simulink model "linear_Plant"  (Simulink 8.1)
settings: Solver=ode4  StartTime=0.0  StopTime=10  FixedStep=0.001  RelTol=1e-3
values from neighbouring files (symbols this model uses):
  a_m = -4    [MRAC_script.m]
  a_p = 1    [MRAC_script.m]
  Gamma = eye(6)*2    [MRAC_script.m]
  k_m = 4    [MRAC_script.m]
  k_p = 3    [MRAC_script.m]
  k_star = k_m/k_p    (= 1.33333333333)    [MRAC_script.m]
  param_0 = [0 0 0 0 0 0]    [MRAC_script.m]
  theta_star = (a_m-a_p)/k_p    (= -1.66666666667)    [MRAC_script.m]
  x_m_0 = 0    [MRAC_script.m]
  x_p_0 = 0    [MRAC_script.m]
settings Model: Creator=patrick  LastModifiedBy=patrick
settings DataIOCC: SignalLoggingSaveFormat=Dataset
settings OptimizationCC: ExpressionDepthLimit=128
settings DebuggingCC: UnderspecifiedInitializationDetection=Simplified  FcnCallInpInsideContextMsg=EnableAllAsError  StateNameClashWarn=none
settings GRTTargetCC: CodeReplacementLibrary=C89/C90 (ANSI)  CombineOutputUpdateFcns=on  GRTInterface=off

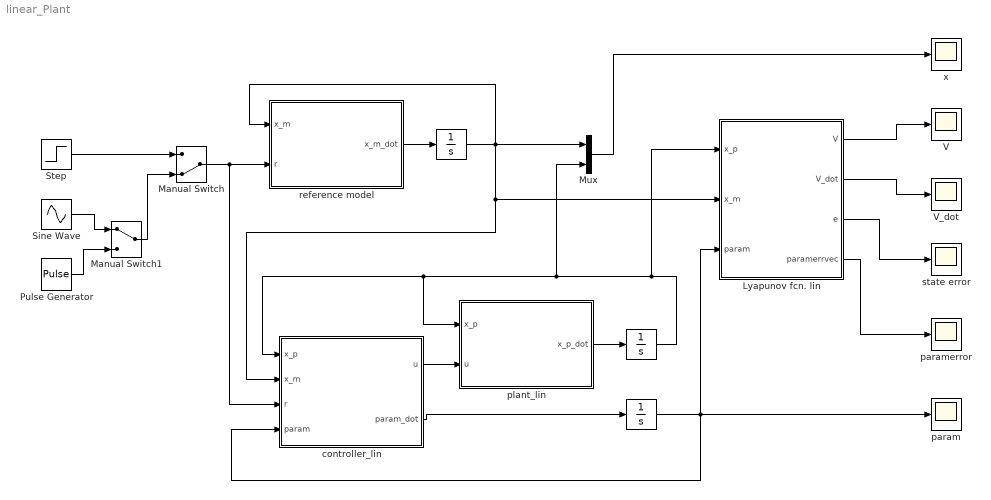
== system linear_Plant ==
  " " : Integrator  InitialCondition=x_p_0
  "    " : Integrator  InitialCondition=param_0(1:2)'
  "     " : Integrator  InitialCondition=x_m_0
  Lyapunov fcn. lin : MATLAB Function  TreatAsAtomicUnit=on
      settings: PermitHierarchicalResolution=ParametersOnly
  Manual Switch : ManualSwitch  CurrentSetting=0
  Manual Switch1 : ManualSwitch
  Mux : Mux  Inputs=2
  Pulse Generator : DiscretePulseGenerator  PulseType=Time based  Amplitude=4  Period=4  PulseWidth=50
  Sine Wave : Sin  Amplitude=4  Frequency=2*pi/4  SampleTime=0
  Step : Step  SampleTime=0
  V : Scope
      settings: SaveName=lyapunov
  "V_dot " : Scope
      settings: SaveName=lyapunov_dot
  controller_lin : MATLAB Function  TreatAsAtomicUnit=on
      settings: PermitHierarchicalResolution=ParametersOnly
  param : Scope
      settings: SaveName=parameters
  paramerror : Scope
      settings: SaveName=parameter_errors
  plant_lin : MATLAB Function  TreatAsAtomicUnit=on
      settings: PermitHierarchicalResolution=ParametersOnly
  reference model : MATLAB Function  TreatAsAtomicUnit=on
      settings: PermitHierarchicalResolution=ParametersOnly
  "state error " : Scope
      settings: SaveName=error
  x : Scope
      settings: SaveName=modelAndPlant
  wires:
  controller_lin/1(u) -> plant_lin/2(u)
  reference model/1(x_m_dot) -> "     "/1
  plant_lin/1(x_p_dot) -> " "/1
  " "/1 -> Lyapunov fcn. lin/1(x_p), Mux/2, plant_lin/1(x_p), controller_lin/1(x_p)
  Step/1 -> Manual Switch/1
  Manual Switch1/1 -> Manual Switch/2
  Sine Wave/1 -> Manual Switch1/1
  Pulse Generator/1 -> Manual Switch1/2
  "     "/1 -> Mux/1, controller_lin/2(x_m), Lyapunov fcn. lin/2(x_m), reference model/1(x_m)
  controller_lin/2(param_dot) -> "    "/1
  Mux/1 -> x/1
  Manual Switch/1 -> controller_lin/3(r), reference model/2(r)
  Lyapunov fcn. lin/1(V) -> V/1
  Lyapunov fcn. lin/2(V_dot) -> "V_dot "/1
  Lyapunov fcn. lin/4(paramerrvec) -> paramerror/1
  "    "/1 -> param/1, controller_lin/4(param), Lyapunov fcn. lin/3(param)
  Lyapunov fcn. lin/3(e) -> "state error "/1

== matlab function reference model ==
  data: x_m_dot output double; x_m input double; r input double; a_m parameter double; k_m parameter double
function x_m_dot = reference_model(x_m, r, a_m, k_m)

x_m_dot=a_m*x_m+k_m*r;      %reference model dynamics with parameters from script

end

== matlab function controller_lin ==
  data: u output double; x_p input double; x_m input double; k_p parameter double; r input double; param input double; param_dot output double; Gamma parameter double
function [u, param_dot] = controller_lin(x_p, x_m, k_p, r, param, Gamma)

e=x_p-x_m;                                            %error

regressor=[x_p; r];                                   %regressor vector

param_dot=-sign(k_p)*Gamma(1:2,1:2)*regressor*e;      %adaptive law

u=param'*regressor;                                   %control signal

end

== matlab function plant_lin ==
  data: x_p_dot output double; x_p input double; a_p parameter double; k_p parameter double; u input double
function x_p_dot = plant_lin(x_p, a_p, k_p,u)

x_p_dot=a_p*x_p+k_p*u;          %plant dynamics with parameters from script

end

== matlab function Lyapunov fcn. lin ==
  data: V output double; x_p input double; x_m input double; theta_star parameter double; k_star parameter double; k_p parameter double; a_m parameter double; Gamma parameter double; param input double; V_dot output double; e output double; paramerrvec output double
function [V, V_dot, e, paramerrvec ] = lyapunov_fcn_lin(x_p, x_m, theta_star, k_star, k_p, a_m, Gamma,  param)

e=x_p-x_m;                          %state error

param_star=[theta_star, k_star];    %true parameters read from script stored in vector

paramerrvec=param-param_star';      %parameter errorvector

V=0.5*e^2+0.5*abs(k_p)*(paramerrvec'*Gamma(1:2,1:2)^-1*paramerrvec);    %Lyapunov function

V_dot=a_m*e^2;                                                          %Lyapunov function derrivative

end
